simulink model "Block_Diagram_open_loop_controlled"  (R2016a)
settings: Solver=VariableStepAuto  StartTime=0.0  StopTime=50  RelTol=1e-3
settings Model: Creator=Muhammad Zubair  LastModifiedBy=Muhammad Zubair

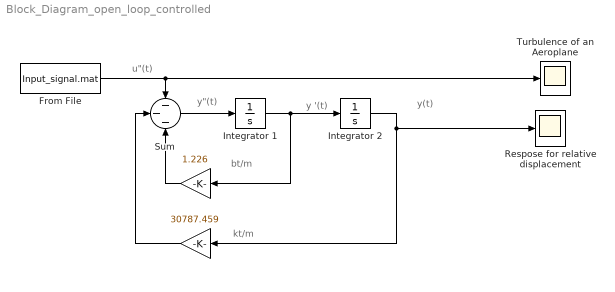
== system Block_Diagram_open_loop_controlled ==
  note: u"(t)
  note: kt/m
  note: bt/m
  note: y(t)
  note: y '(t)
  note: y"(t)
  " " : Gain  Gain=1.226
  "  " : Gain  Gain=30787.459
  From File : FromFile  FileName=Input_signal.mat  SampleTime=0
  Integrator 1 : Integrator
  "Integrator 2 " : Integrator
  Respose for relative displacement : Scope
  Sum : Sum  Inputs=---
  Turbulence of an Aeroplane : Scope
  wires:
  Integrator 1/1 -> " "/1, "Integrator 2 "/1
  "Integrator 2 "/1 -> Respose for relative displacement/1, "  "/1
  From File/1 -> Turbulence of an Aeroplane/1, Sum/1
  "  "/1 -> Sum/2
  " "/1 -> Sum/3
  Sum/1 -> Integrator 1/1
